simulink subsystem "power_window_system_impact_V6"  (R2021a)
settings: Solver=VariableStepAuto  StartTime=0.0  StopTime=10.0  RelTol=1e-3
settings Model: Creator=achu  LastModifiedBy=achu

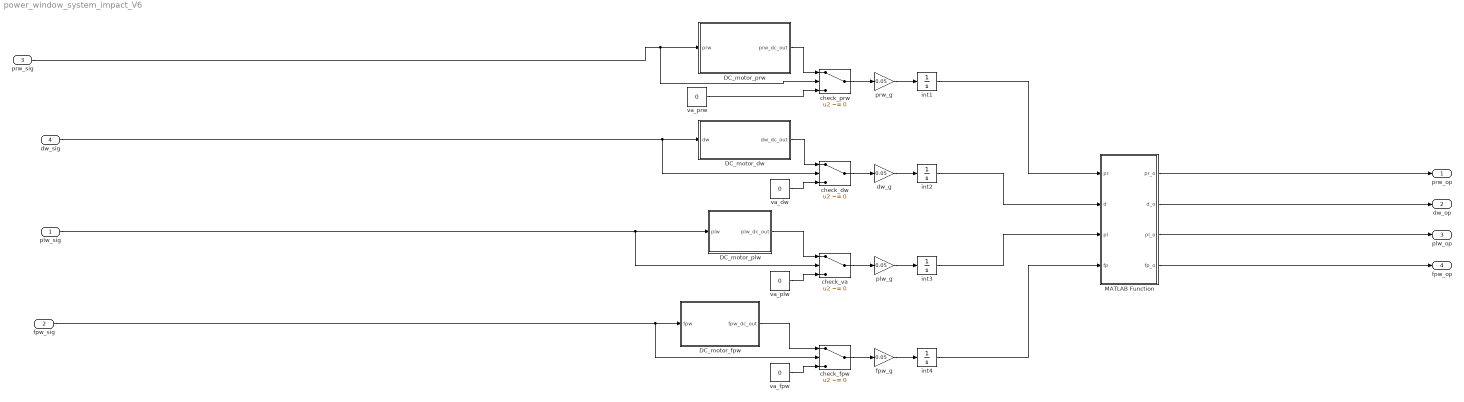
== system power_window_system_impact_V6 ==
  plw_sig : Inport
  fpw_sig : Inport  Port=2
  prw_sig : Inport  Port=3
  dw_sig : Inport  Port=4
  DC_motor_dw : Subsystem
  DC_motor_fpw : Subsystem
  DC_motor_plw : Subsystem
  DC_motor_prw : Subsystem
  MATLAB Function : MATLAB Function  TreatAsAtomicUnit=on
  check_dw : Switch  Criteria=u2 ~= 0
  check_fpw : Switch  Criteria=u2 ~= 0
  check_prw : Switch  Criteria=u2 ~= 0
  check_va : Switch  Criteria=u2 ~= 0
  dw_g : Gain  Gain=0.05
  fpw_g : Gain  Gain=0.05
  int{1..4} (4 alike) : Integrator  InitialCondition=0.0001
      settings: AttributesFormatString=%<InitialCondition>
  plw_g : Gain  Gain=0.05
  prw_g : Gain  Gain=0.05
  va_dw : Constant  Value=0
  va_fpw : Constant  Value=0
  va_plw : Constant  Value=0
  va_prw : Constant  Value=0
  prw_op : Outport
  dw_op : Outport  Port=2
  plw_op : Outport  Port=3
  fpw_op : Outport  Port=4
  wires:
  fpw_sig/1 -> DC_motor_fpw/1(fpw), check_fpw/2
  dw_sig/1 -> check_dw/2, DC_motor_dw/1(dw)
  va_plw/1 -> check_va/3
  check_va/1 -> plw_g/1
  va_prw/1 -> check_prw/3
  DC_motor_plw/1(plw_dc_out) -> check_va/1
  dw_g/1 -> int2/1
  int4/1 -> MATLAB Function/4(fp)
  int3/1 -> MATLAB Function/3(pl)
  check_fpw/1 -> fpw_g/1
  check_dw/1 -> dw_g/1
  DC_motor_prw/1(prw_dc_out) -> check_prw/1
  va_fpw/1 -> check_fpw/3
  check_prw/1 -> prw_g/1
  int2/1 -> MATLAB Function/2(d)
  fpw_g/1 -> int4/1
  plw_g/1 -> int3/1
  MATLAB Function/1(pr_o) -> prw_op/1
  int1/1 -> MATLAB Function/1(pr)
  prw_sig/1 -> DC_motor_prw/1(prw), check_prw/2
  prw_g/1 -> int1/1
  va_dw/1 -> check_dw/3
  plw_sig/1 -> check_va/2, DC_motor_plw/1(plw)
  DC_motor_dw/1(dw_dc_out) -> check_dw/1
  MATLAB Function/2(d_o) -> dw_op/1
  MATLAB Function/3(pl_o) -> plw_op/1
  MATLAB Function/4(fp_o) -> fpw_op/1
  DC_motor_fpw/1(fpw_dc_out) -> check_fpw/1

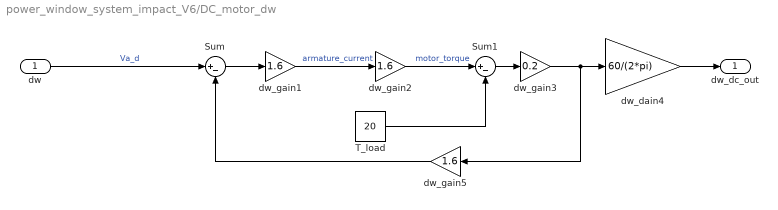
== system power_window_system_impact_V6/DC_motor_dw ==
  dw : Inport
  Sum : Sum  Inputs=|+-
  Sum1 : Sum  Inputs=|+-
  T_load : Constant  Value=20
  dw_dain4 : Gain  Gain=60/(2*pi)
  dw_gain1 : Gain  Gain=1.6
  dw_gain2 : Gain  Gain=1.6
  dw_gain3 : Gain  Gain=0.2
  dw_gain5 : Gain  Gain=1.6
  dw_dc_out : Outport
  wires:
  dw/1 -> Sum/1  "Va_d"
  dw_gain3/1 -> dw_dain4/1, dw_gain5/1
  T_load/1 -> Sum1/2
  dw_gain1/1 -> dw_gain2/1  "armature_current"
  dw_gain5/1 -> Sum/2
  dw_dain4/1 -> dw_dc_out/1
  Sum/1 -> dw_gain1/1
  Sum1/1 -> dw_gain3/1
  dw_gain2/1 -> Sum1/1  "motor_torque"

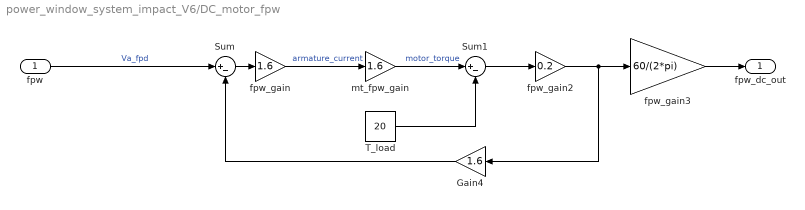
== system power_window_system_impact_V6/DC_motor_fpw ==
  fpw : Inport
  Gain4 : Gain  Gain=1.6
  Sum : Sum  Inputs=|+-
  Sum1 : Sum  Inputs=|+-
  T_load : Constant  Value=20
  fpw_gain : Gain  Gain=1.6
  fpw_gain2 : Gain  Gain=0.2
  fpw_gain3 : Gain  Gain=60/(2*pi)
  mt_fpw_gain : Gain  Gain=1.6
  fpw_dc_out : Outport
  wires:
  fpw/1 -> Sum/1  "Va_fpd"
  fpw_gain2/1 -> fpw_gain3/1, Gain4/1
  T_load/1 -> Sum1/2
  fpw_gain/1 -> mt_fpw_gain/1  "armature_current"
  Gain4/1 -> Sum/2
  fpw_gain3/1 -> fpw_dc_out/1
  Sum/1 -> fpw_gain/1
  Sum1/1 -> fpw_gain2/1
  mt_fpw_gain/1 -> Sum1/1  "motor_torque"

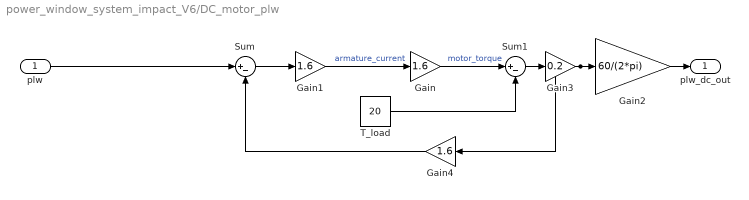
== system power_window_system_impact_V6/DC_motor_plw ==
  plw : Inport
  Gain : Gain  Gain=1.6
  Gain1 : Gain  Gain=1.6
  Gain2 : Gain  Gain=60/(2*pi)
  Gain3 : Gain  Gain=0.2
  Gain4 : Gain  Gain=1.6
  Sum : Sum  Inputs=|+-
  Sum1 : Sum  Inputs=|+-
  T_load : Constant  Value=20
  plw_dc_out : Outport
  wires:
  plw/1 -> Sum/1
  Gain3/1 -> Gain2/1, Gain4/1
  T_load/1 -> Sum1/2
  Gain1/1 -> Gain/1  "armature_current"
  Gain4/1 -> Sum/2
  Gain2/1 -> plw_dc_out/1
  Sum/1 -> Gain1/1
  Sum1/1 -> Gain3/1
  Gain/1 -> Sum1/1  "motor_torque"

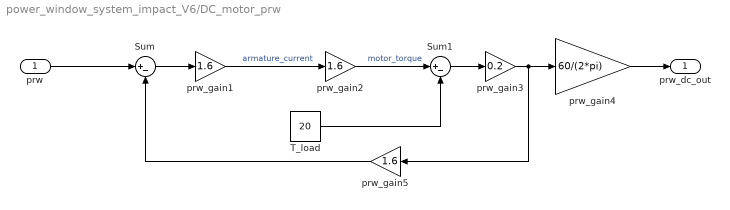
== system power_window_system_impact_V6/DC_motor_prw ==
  prw : Inport
  Sum : Sum  Inputs=|+-
  Sum1 : Sum  Inputs=|+-
  T_load : Constant  Value=20
  prw_gain1 : Gain  Gain=1.6
  prw_gain2 : Gain  Gain=1.6
  prw_gain3 : Gain  Gain=0.2
  prw_gain4 : Gain  Gain=60/(2*pi)
  prw_gain5 : Gain  Gain=1.6
  prw_dc_out : Outport
  wires:
  prw/1 -> Sum/1
  prw_gain3/1 -> prw_gain4/1, prw_gain5/1
  T_load/1 -> Sum1/2
  prw_gain1/1 -> prw_gain2/1  "armature_current"
  prw_gain5/1 -> Sum/2
  prw_gain4/1 -> prw_dc_out/1
  Sum/1 -> prw_gain1/1
  Sum1/1 -> prw_gain3/1
  prw_gain2/1 -> Sum1/1  "motor_torque"

== matlab function power_window_system_impact_V6/MATLAB Function ==
  data: pr input; pr_o output; d input; pl input; fp input; d_o output; pl_o output; fp_o output
function [pr_o,d_o, pl_o, fp_o] = fcn(pr, d, pl, fp)
if pr>=10
    prout=10;
elseif pr<=0
    prout=0;
else
    prout=pr;
end

if d>=10
    dout=10;
elseif d<=0
    dout=0;
else
    dout=d;
end

if pl>=10
    plout=10;
elseif pl<=0
    plout=0;
else
    plout=pr;
end

if fp>=10
    fpout=10;
elseif fp<=0
    fpout=0;
else
    fpout=fp;
end
pr_o=prout;
d_o=dout;
pl_o=plout;
fp_o=fpout;
